simulink model "CartesianPosControl5bar"  (R2018b)
settings: Solver=VariableStepAuto  StartTime=0.0  StopTime=10  RelTol=1e-3
undefined symbols (not defined in the file): x, y
libraries: simulink x2
settings Model: Creator=Srikar  LastModifiedBy=holyCow
settings SFSimCC: SimUseLocalCustomCode=off
settings RTWCC: RTWUseLocalCustomCode=off

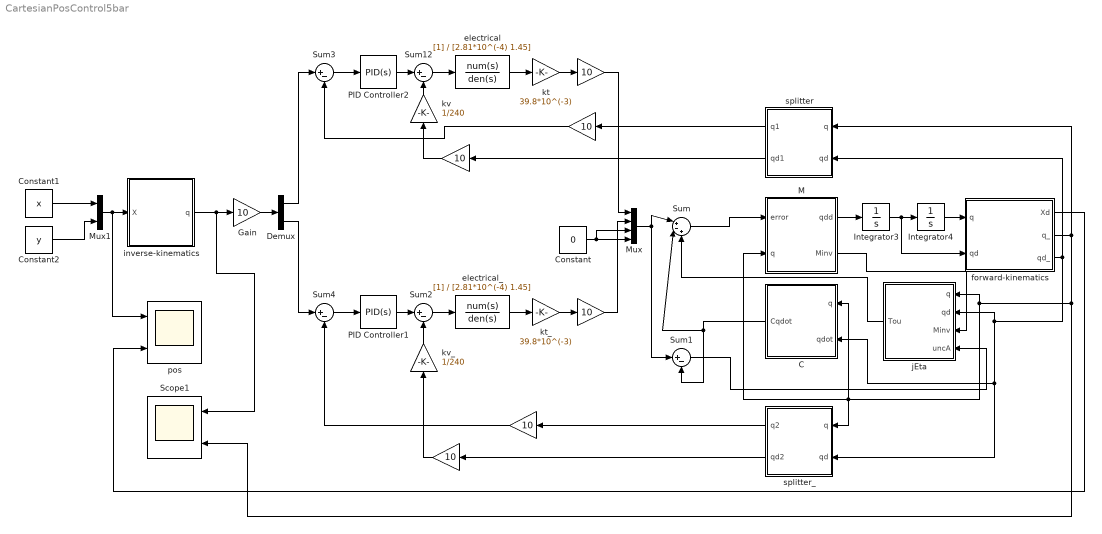
== system CartesianPosControl5bar ==
  " " : Gain  Gain=10
  "  " : Gain  Gain=10
  "   " : Gain  Gain=10
  "    " : Gain  Gain=10
  "         " : Gain  Gain=10
  "                  " : Gain  Gain=10
  C : MATLAB Function  TreatAsAtomicUnit=on
  Constant : Constant  Value=0
  Constant1 : Constant  Value=x
  Constant2 : Constant  Value=y
  Demux : Demux  Outputs=2
  Gain : Gain  Gain=10
  Integrator3 : Integrator  InitialCondition=[0 0 0 0]'
  Integrator4 : Integrator  InitialCondition=[0 0 0 0]'
  M : MATLAB Function  TreatAsAtomicUnit=on
  Mux : Mux
  Mux1 : Mux  Inputs=2
  PID Controller1 : simulink/Continuous/PID Controller  Controller=PID  Form=Parallel  TimeDomain=Continuous-time  SampleTime=-1  IntegratorMethod=Forward Euler  FilterMethod=Forward Euler  ControllerParametersSource=internal  P=4.03915691539375  I=47.1446499264724  D=0.0745984943668176  UseFilter=on  N=1888.25178733024  TunerSelectOption=Transfer Function Based (PID Tuner App)  InitialConditionSource=internal  InitialConditionForIntegrator=0  InitialConditionForFilter=0  DifferentiatorICPrevScaledInput=0  ExternalReset=none  TrackingMode=off  Kt=1  LimitOutput=off  UpperSaturationLimit=inf  LowerSaturationLimit=-inf  LinearizeAsGain=on  AntiWindupMode=none  Kb=1  POutMin=[]  POutMax=[]  IOutMin=[]  IOutMax=[]  DOutMin=[]  DOutMax=[]  NOutMin=[]  NOutMax=[]  SumOutMin=[]  SumOutMax=[]  SaturationOutMin=[]  SaturationOutMax=[]  PParamMin=[]  PParamMax=[]  IParamMin=[]  IParamMax=[]  DParamMin=[]  DParamMax=[]  NParamMin=[]  NParamMax=[]  KbParamMin=[]  KbParamMax=[]  KtParamMin=[]  KtParamMax=[]  KbOutMin=[]  KbOutMax=[]  KtOutMin=[]  KtOutMax=[]  IntegratorOutMin=[]  IntegratorOutMax=[]  FilterOutMin=[]  FilterOutMax=[]  SumI1OutMin=[]  SumI1OutMax=[]  SumI2OutMin=[]  SumI2OutMax=[]  SumI3OutMin=[]  SumI3OutMax=[]  SumI4OutMin=[]  SumI4OutMax=[]  SumDOutMin=[]  SumDOutMax=[]  DifferentiatorOutMin=[]  DifferentiatorOutMax=[]  FilterDiffOutCoefMin=[]  FilterDiffOutCoefMax=[]  ReciprocalOutMin=[]  ReciprocalOutMax=[]  SumDenOutMin=[]  SumDenOutMax=[]  SumNumOutMin=[]  SumNumOutMax=[]  DivideOutMin=[]  DivideOutMax=[]  IntegratorContinuousStateAttributes=''  IntegratorStateMustResolveToSignalObject=off  IntegratorRTWStateStorageClass=Auto  FilterContinuousStateAttributes=''  FilterStateMustResolveToSignalObject=off  FilterRTWStateStorageClass=Auto  ParallelPVariant=InternalParameters  IdealPVariant=Disabled  IVariant=InternalParameters  DVariant=InternalParameters  IntegratorVariant=Continuous  SatVariant=Disabled  AWVariant=Passthrough  PCopyVariant=Disabled  TRVariant=Disabled  FdbkBlocksVariant=Forward  IdealPFdbkVariant=Disabled  SatFdbkVariant=Disabled  DerivativeFilterVariant=ContFilter  NVariant=InternalParameters  NCopyVariant=Disabled  FilterICVariant=InternalICsFilter  IntegratorICVariant=InternalICs  ExternalResetVariant=Disabled  TRSumVariant=Passthrough  SumFdbkVariant=Disabled  SumVariant=Sum_PID
  PID Controller2 : simulink/Continuous/PID Controller  Controller=PID  Form=Parallel  TimeDomain=Continuous-time  SampleTime=-1  IntegratorMethod=Forward Euler  FilterMethod=Forward Euler  ControllerParametersSource=internal  P=4.03915691539375  I=47.1446499264724  D=0.0745984943668176  UseFilter=on  N=1888.25178733024  TunerSelectOption=Transfer Function Based (PID Tuner App)  InitialConditionSource=internal  InitialConditionForIntegrator=0  InitialConditionForFilter=0  DifferentiatorICPrevScaledInput=0  ExternalReset=none  TrackingMode=off  Kt=1  LimitOutput=off  UpperSaturationLimit=inf  LowerSaturationLimit=-inf  LinearizeAsGain=on  AntiWindupMode=none  Kb=1  POutMin=[]  POutMax=[]  IOutMin=[]  IOutMax=[]  DOutMin=[]  DOutMax=[]  NOutMin=[]  NOutMax=[]  SumOutMin=[]  SumOutMax=[]  SaturationOutMin=[]  SaturationOutMax=[]  PParamMin=[]  PParamMax=[]  IParamMin=[]  IParamMax=[]  DParamMin=[]  DParamMax=[]  NParamMin=[]  NParamMax=[]  KbParamMin=[]  KbParamMax=[]  KtParamMin=[]  KtParamMax=[]  KbOutMin=[]  KbOutMax=[]  KtOutMin=[]  KtOutMax=[]  IntegratorOutMin=[]  IntegratorOutMax=[]  FilterOutMin=[]  FilterOutMax=[]  SumI1OutMin=[]  SumI1OutMax=[]  SumI2OutMin=[]  SumI2OutMax=[]  SumI3OutMin=[]  SumI3OutMax=[]  SumI4OutMin=[]  SumI4OutMax=[]  SumDOutMin=[]  SumDOutMax=[]  DifferentiatorOutMin=[]  DifferentiatorOutMax=[]  FilterDiffOutCoefMin=[]  FilterDiffOutCoefMax=[]  ReciprocalOutMin=[]  ReciprocalOutMax=[]  SumDenOutMin=[]  SumDenOutMax=[]  SumNumOutMin=[]  SumNumOutMax=[]  DivideOutMin=[]  DivideOutMax=[]  IntegratorContinuousStateAttributes=''  IntegratorStateMustResolveToSignalObject=off  IntegratorRTWStateStorageClass=Auto  FilterContinuousStateAttributes=''  FilterStateMustResolveToSignalObject=off  FilterRTWStateStorageClass=Auto  ParallelPVariant=InternalParameters  IdealPVariant=Disabled  IVariant=InternalParameters  DVariant=InternalParameters  IntegratorVariant=Continuous  SatVariant=Disabled  AWVariant=Passthrough  PCopyVariant=Disabled  TRVariant=Disabled  FdbkBlocksVariant=Forward  IdealPFdbkVariant=Disabled  SatFdbkVariant=Disabled  DerivativeFilterVariant=ContFilter  NVariant=InternalParameters  NCopyVariant=Disabled  FilterICVariant=InternalICsFilter  IntegratorICVariant=InternalICs  ExternalResetVariant=Disabled  TRSumVariant=Passthrough  SumFdbkVariant=Disabled  SumVariant=Sum_PID
  Scope1 : Scope  NumInputPorts=2
  Sum : Sum  Inputs=|+-+
  Sum{1..4,12} (5 alike) : Sum  Inputs=|+-
  electrical : TransferFcn  Denominator=[2.81*10^(-4) 1.45]
  electrical_ : TransferFcn  Denominator=[2.81*10^(-4) 1.45]
  forward-kinematics : MATLAB Function  TreatAsAtomicUnit=on
  inverse-kinematics : MATLAB Function  TreatAsAtomicUnit=on
  jEta : MATLAB Function  TreatAsAtomicUnit=on
  kt : Gain  Gain=39.8*10^(-3)
  kt_ : Gain  Gain=39.8*10^(-3)
  kv : Gain  Gain=1/240
  kv_ : Gain  Gain=1/240
  pos : Scope  NumInputPorts=2
  splitter : MATLAB Function  TreatAsAtomicUnit=on
  splitter_ : MATLAB Function  TreatAsAtomicUnit=on
  wires:
  Constant/1 -> Mux/3, Mux/4
  "  "/1 -> kv/1
  electrical/1 -> kt/1
  PID Controller2/1 -> Sum12/1
  " "/1 -> Sum3/2
  kv/1 -> Sum12/2
  Sum12/1 -> electrical/1
  kt/1 -> "                  "/1
  Sum3/1 -> PID Controller2/1
  "                  "/1 -> Mux/1
  splitter/1(q1) -> " "/1
  splitter/2(qd1) -> "  "/1
  "   "/1 -> Sum4/2
  kt_/1 -> "         "/1
  electrical_/1 -> kt_/1
  Sum2/1 -> electrical_/1
  "    "/1 -> kv_/1
  kv_/1 -> Sum2/2
  PID Controller1/1 -> Sum2/1
  Sum4/1 -> PID Controller1/1
  "         "/1 -> Mux/2
  splitter_/1(q2) -> "   "/1
  splitter_/2(qd2) -> "    "/1
  forward-kinematics/1(Xd) -> pos/2
  forward-kinematics/3(qd_) -> splitter_/2(qd), C/2(qdot), jEta/2(qd), splitter/2(qd)
  Integrator4/1 -> forward-kinematics/1(q)
  forward-kinematics/2(q_) -> splitter/1(q), Scope1/2, splitter_/1(q), C/1(q), M/2(q), jEta/1(q)
  M/1(qdd) -> Integrator3/1
  Sum/1 -> M/1(error)
  Sum1/1 -> jEta/4(uncA)
  C/1(Cqdot) -> Sum/2, Sum1/2
  M/2(Minv) -> jEta/3(Minv)
  jEta/1(Tou) -> Sum/3
  Mux/1 -> Sum/1, Sum1/1
  Integrator3/1 -> forward-kinematics/2(qd), Integrator4/1
  Constant1/1 -> Mux1/1
  Constant2/1 -> Mux1/2
  Mux1/1 -> pos/1, inverse-kinematics/1(X)
  inverse-kinematics/1(q) -> Scope1/1, Gain/1
  Gain/1 -> Demux/1
  Demux/1 -> Sum3/1
  Demux/2 -> Sum4/1

== matlab function CartesianPosControl5bar/splitter ==
  data: q input; q1 output; qd input; qd1 output
function [q1, qd1] = fcn(q, qd)
q1 = q(1);
qd1 = qd(1);

== matlab function CartesianPosControl5bar/inverse-kinematics ==
  data: X input; q output
function q = fcn(X)
l = 0.18;
b = 0.155;
x = X(1);
y = X(2);

m = sqrt(x^2 + y^2); %pa1
n = sqrt((x-b)^2 + y^2); %pa2

q21 = acos(m/(2*l));
q22 = acos(x/m);
q2 = q21 + q22;

q11 = acos(n/(2*l));
q12 = acos((x-b)/n);
q1 = q12 - q11;

q = [q1; q2];

== matlab function CartesianPosControl5bar/C ==
  data: q input; Cqdot output; qdot input
function Cqdot  = fcn(q, qdot)
q1 = q(1);
q2 = q(2);
q3 = q(3);
q4 = q(4);

C=[0.E-307,(-0.234804E-3).*cos(q1).*sin(q2),0.496696E-3.*sin(q1+(-1).*q3),cos(q1).*((-0.234804E-3).*sin(q1)+(-0.234804E-3).*sin(q2));0.234804E-3.*cos(q1).*sin(q2),0.E-307,0,0.234804E-3.*cos(q1).*sin(q2)+(-0.469609E-3).*cos(q2).*sin(q4);(-0.496696E-3).*sin(q1+(-1).*q3),0,0.E-307,0;cos(q1).*(0.234804E-3.*sin(q1)+0.234804E-3.*sin(q2)),0.469609E-3.*cos(q2).*sin(q1)+(0.234804E-3.*cos(q1)+(-0.469609E-3).*cos(q4)).*sin(q2),0,0.234804E-3.*cos(q1).*sin(q1)+(-0.234804E-3).*cos(q4).*sin(q4)];
Cqdot = C*qdot;

== matlab function CartesianPosControl5bar/splitter_ ==
  data: q input; q2 output; qd input; qd2 output
function [q2, qd2] = fcn(q, qd)
q2 = q(2);
qd2 = qd(2);

== matlab function CartesianPosControl5bar/jEta ==
  data: Tou output; q input; qd input; Minv input; uncA input
function Tou  = fcn(q, qd, Minv, uncA)
l = 0.18;
q1 = q(1);
q2 = q(2);
q3 = q(3);
q4 = q(4);

JEta = l .* [sin(q1) -sin(q2) sin(q3) -sin(q4);
                -cos(q1) cos(q2) -cos(q3) cos(q4)];
   
Jdot = l .* [cos(q1) -cos(q2) cos(q3) -cos(q4)
                sin(q1) -sin(q2) sin(q3) -sin(q4)];

B = (JEta * Minv * uncA) + (Jdot * qd);
A = inv(JEta * Minv * JEta');
lambda = -1 * (A * B);

Tou = JEta' * lambda;

== matlab function CartesianPosControl5bar/M ==
  data: error input; qdd output; q input; Minv output
function [qdd, Minv]  = fcn(error, q)
l=0.18;
q1 = q(1);
q2 = q(2);
q3 = q(3);
q4 = q(4);

m1=0.03285303;
m2=0.02898819;
m3=0.03066024;
m4=0.02898819;
I1=2.19e-006;
I2=1.99e-006;
I3=1.2e-006;
I4=1.99e-006;
Jv1=[(-l/2)*sin(q1) 0 0 0; (l/2)*cos(q1) 0 0 0];
Jv2=[0 (-l/2)*sin(q2) 0 0; 0 (l/2)*cos(q2) 0 0];
Jv3=[-l*sin(q1) 0 (-l/2)*sin(q3) 0; l*cos(q1) 0 (l/2)*cos(q3) 0];
Jv4=[0 -l*sin(q2) 0 (-l/2)*sin(q4); 0 l*cos(q2) 0 (l/2)*cos(q4)];
Jw1=[0 0 0 0;0 0 0 0;1 0 0 0];
Jw2=[0 0 0 0;0 0 0 0;0 1 0 0];
Jw3=[0 0 0 0;0 0 0 0;0 0 1 0];
Jw4=[0 0 0 0;0 0 0 0;0 0 0 1];
M=(Jv1')*m1*(Jv1)+(Jv2')*m2*(Jv2)+(Jv3')*m3*(Jv3)+(Jv4')*m4*(Jv4)+(Jw1')*I1*(Jw1)+(Jw2')*I2*(Jw2)+(Jw3')*I3*(Jw3)+(Jw4')*I4*(Jw4);
% M = (Jw1')*I1*(Jw1)+(Jw2')*I2*(Jw2)+(Jw3')*I3*(Jw3)+(Jw4')*I4*(Jw4);
% M = [1 0 0 0; 0 1 0 0; 0 0 1 0; 0 0 0 1];
Minv=inv(M);
qdd = Minv * error;

== matlab function CartesianPosControl5bar/forward-kinematics ==
  data: q input; Xd output; q_ output; qd_ output; qd input
function [Xd, q_, qd_]  = fcn(q, qd)

q1 = q(1);
q2 = q(2);

l = 0.18;
b = 0.155;

xb = l*cos(q2);
yb = l*sin(q2);
xd = b + l*cos(q1);
yd = l*sin(q1);

dsquare = (xb - xd)^2 + (yb - yd)^2;

%by Heron's formula
k = 0.25 * sqrt(((2*l)^2 - dsquare) * (dsquare));

%considering only the y-coordinate that is above the line joining the
%centers of the corresponding two circles.
x = (0.5 * (xb + xd)) + (2 * (yb - yd) * (k/dsquare));
y = (0.5 * (yb + yd)) + (2 * (xd - xb) * (k/dsquare));

%now for computing q3 and q4,
q4 = asin((y - (l*sin(q2)))/l);
q3 = acos((x - b - l*cos(q1))/l);

%for q3d and q4d,
a = sin(q2)*qd(2) - sin(q1)*qd(1);
b = cos(q1)*qd(1) - cos(q2)*qd(2);
c = sin(q3)*cos(q4) - sin(q4)*cos(q3);

q3d = (cos(q4)*a + sin(q4)*b)/c;
q4d = (sin(q3)*q3d + sin(q1)*qd(1) - sin(q2)*qd(2))/sin(q4);

q_ = [q1; q2; q3; q4];
qd_ = [qd(1); qd(2); q3d; q4d];

Xd = [x; y];
